simulink library "AddOn_Lib_TTC580_CCP"  (R2021a)
settings: Solver=VariableStepAuto  StartTime=0.0  StopTime=10.0  RelTol=1e-3
PreLoadFcn:
  | addpath(genpath(fileparts(which('AddOn_Lib_TTC580_CCP'))));
  | try
  | addpath([fileparts(which('AddOn_Lib_TTC580_CCP')),'\..\CustomClasses']);
  | catch
  | warning('AddOn_Lib_TTC580: add path to CustomClasses manually');
  | end
undefined symbols (not defined in the file): IO_Blk_Lib_TTC500, MainDlg_basic, MainDlg_CCP_J1939_
(part 3 of 3)

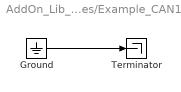
== system AddOn_Lib_TTC580_CCP/Examples/Example_CAN1 ==
  Ground : Ground
  Terminator : Terminator
  wires:
  Ground/1 -> Terminator/1

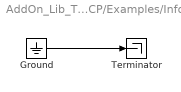
== system AddOn_Lib_TTC580_CCP/Examples/Info ==
  Ground : Ground
  Terminator : Terminator
  wires:
  Ground/1 -> Terminator/1

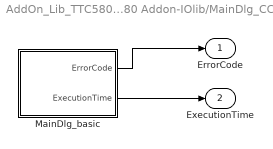
== system AddOn_Lib_TTC580_CCP/System  Blocks TTC580 Addon-IOlib/MainDlg_CCP ==
  MainDlg_basic : Subsystem  Priority=-2147483646  LoadFcn=|  mask(MainDlg_basic_Code){SampleTime=-1, ttlib=IO_Blk_Lib_TTC500, ttDescription=MainDlg_basic, tt_iolib_version=0.25, baudrate_CAN0=baudrate_CAN0, tseg1_CAN0=tseg1_CAN0, tseg2_CAN0=tseg2_CAN0, sjw_CAN0=sjw_CAN0, brp_CAN0=brp_CAN0, baudrate_CAN1=baudrate_CAN1, tseg1_CAN1=tseg1_CAN1, tseg2_CAN1=tseg2_CAN1, sjw_CAN1=sjw_CAN1, brp_CAN1=brp_CAN1, baudrate_CAN2=baudrate_CAN2, tseg1_CAN2=tseg1_CAN2, tseg2_CAN2=tseg2_CAN2, sjw_CAN2=sjw_CAN2, brp_CAN2=brp_CAN2, baudrate_CAN3=baudrate_CAN3, baudrate_CAN4=baudrate_CAN4, baudrate_CAN5=baudrate_CAN5, baudrate_CAN6=baudrate_CAN6, tseg1=tseg1, tseg2=tseg2, sjw=sjw, Duration_ms=Duration_ms, glitch_filter_time=glitch_filter_time, watchdog_window_size=watchdog_window_size, watchdog_reset_behavior=watchdog_reset_behavior, brp=brp, Major_Number=Major_Number, Minor_Number=Minor_Number, Revison_Number=Revison_Number, Node_Number=Node_Number, Enable_Reset_by_TTCDownloader=Enable_Reset_by_TTCDownloader, Enable_CCP=Enable_CCP, CRO_ID=CRO_ID, DTO_ID=DTO_ID, CCP_Station_Addr=CCP_Station_Addr, CCP_Station_ID=CCP_Station_ID, CPP_channel=CPP_channel, CPP_id_format=CPP_id_format, bEnable_DAQ0=bEnable_DAQ0, bEnable_DAQ1_2=bEnable_DAQ1_2, ODT_total=ODT_total, bEnable_ErrorCBAction=bEnable_ErrorCBAction, bDIAG_ERR_DISABLE_SSW0=bDIAG_ERR_DISABLE_SSW0, bDIAG_ERR_DISABLE_SSW1=bDIAG_ERR_DISABLE_SSW1, bDIAG_ERR_DISABLE_SSW2=bDIAG_ERR_DISABLE_SSW2, bFlashOverEthernet=bFlashOverEthernet}
      | try
      | %
      | %Upgrade Information - standard BEGIN
      | new_color = 'blue';
      | new_ver = '0.25';
      | act_ver = get_param(gcb,'tt_iolib_version');
      | if not(strcmp(act_ver,new_ver))
      |     disp(['Upgrade block: ',gcb,char(10),'       Version: ',act_ver,' to ',new_ver]);
      |     %switch - case for specific upgrade information e.g. additional parameter required 
      |     %Change appearance and version information
      |     set_param(gcb,'ForegroundColor',new_color);
      |     set_param(gcb,'tt_iolib_version',new_ver);
      | end
      | %Upgrade Information - standard END
      | catch
      | %Standard catch section BEGIN
      | errordlg('An error occurred in a callback of the TTC580-BlockLib. Please open the Diagnostic Viewer for further details');
      | disp(' ');
      | disp('------------------------------------------------------------');
      | disp('An error occurred in a callback of the TTC580-BlockLib.');
      | disp(['Please check the parameters in the mask of ',gcb]);
      | disp('If you do not encounter any violations, then please '); 
      | disp('copy the following lines and report this to support@ttcontrol.com ');
      | disp('<< begin of error message dump >>');
      | disp(['Version of TTC580-BlockLib: ', get_param(gcb,'tt_iolib_version')]);
      | disp(get_param(gcb,'ttDescription'));
      | disp(gcb);
      | x=lasterror;disp(x.message);
      | disp(get_param(gcb,'MaskValues'));
      | disp(version);
      | disp(computer);
      | disp('<< end of error message dump >>');
      | disp('------------------------------------------------------------');
      | disp(' ');
      | %Standard catch section END
      | end
      mask help:
      | Block representing the handler for main environment-settings of the applications to be run on a TTC580.
      | Generation of <model>_main.c
      mask init:
      | %
      settings: CopyFcn=%deleted
      mask Help: No further help available for this block
      mask Callback baudrate_CAN0: %
      mask Callback tseg1_CAN0: %
      mask Callback tseg2_CAN0: %
      mask Callback sjw_CAN0: %
      mask Callback brp_CAN0: %
      mask Callback baudrate_CAN1: %
      mask Callback tseg1_CAN1: %
      mask Callback tseg2_CAN1: %
      mask Callback sjw_CAN1: %
      mask Callback brp_CAN1: %
      mask Callback baudrate_CAN2: %
      mask Callback tseg1_CAN2: %
      mask Callback tseg2_CAN2: %
      mask Callback sjw_CAN2: %
      mask Callback brp_CAN2: %
      mask Callback baudrate_CAN3: %
      mask Callback baudrate_CAN4: %
      mask Callback baudrate_CAN5: %
      mask Callback baudrate_CAN6: %
      mask Callback tseg1: %
      mask Callback tseg2: %
      mask Callback sjw: %
      mask Callback Duration_ms: %
      mask Callback glitch_filter_time: %
      mask Callback watchdog_window_size: %
      mask Callback watchdog_reset_behavior: %
      mask Callback brp: %
      mask Callback Major_Number: %
      mask Callback Minor_Number: %
      mask Callback Revison_Number: %
      mask Callback Node_Number: %
      mask Callback Enable_Reset_by_TTCDownloader: %
      mask Callback Enable_CCP: %
      mask Callback CRO_ID: %
      mask Callback DTO_ID: %
      mask Callback CCP_Station_Addr: %
      mask Callback CCP_Station_ID: %
      mask Callback CPP_channel: %
      mask Callback CPP_id_format: %
      mask Callback bEnable_DAQ0: %
      mask Callback bEnable_DAQ1_2: %
      mask Callback ODT_total: %
      mask Callback bEnable_ErrorCBAction: %
      mask Callback bDIAG_ERR_DISABLE_SSW0: %
      mask Callback bDIAG_ERR_DISABLE_SSW1: %
      mask Callback bDIAG_ERR_DISABLE_SSW2: %
      mask Callback bFlashOverEthernet:
      | try
      | s_ParameterDecision = 'bFlashOverEthernet'; %Deside on this parameter
      | c_ValuesDecision={'on'}; %Positive DescitionValues
      | s_ParameterInvisible = 'Enable_Reset_by_TTCDownloader'; %Make this invisible
      | %trim
      | if ischar(s_ParameterInvisible)%if secttion for compatibility reasons of template
      |     cs_ParameterInvisible = {s_ParameterInvisible};
      | else
      |     cs_ParameterInvisible = s_ParameterInvisible;
      | end
      | s_ParameterDecision = strtrim(s_ParameterDecision);
      | c_ValuesDecision = strtrim(c_ValuesDecision);
      | for j=1:length(cs_ParameterInvisible)
      |   s_ParameterInvisible = strtrim(cs_ParameterInvisible{j});
      |   c_MaskVisibilities=get_param(gcb,'MaskVisibilities');
      |   %check consistency
      |   idx=strmatch(s_ParameterInvisible,get_param(gcb,'MaskNames'),'exact');
      |   c_MaskVisibilities{idx}='on'; %default
      |     for i = 1: length(c_ValuesDecision)
      |         if ~isempty(strmatch(get_param(gcb, s_ParameterDecision), c_ValuesDecision{i},'exact'))
      |            c_MaskVisibilities{idx}='off';
      |         end
      |     end
      |   set_param(gcb,'MaskVisibilities',c_MaskVisibilities);
      | end
      | catch
      | %Standard catch section BEGIN
      | errordlg('An error occurred in a callback of the TTC580-BlockLib. Please open the Diagnostic Viewer for further details');
      | disp(' ');
      | disp('------------------------------------------------------------');
      | disp('An error occurred in a callback of the TTC580-BlockLib.');
      | disp(['Please check the parameters in the mask of ',gcb]);
      | disp('If you do not encounter any violations, then please ');
      | disp('copy the following lines and report this to support@ttcontrol.com ');
      | disp('<< begin of error message dump >>');
      | disp(['Version of TTC580-BlockLib: ', get_param(gcb,'tt_iolib_version')]);
      | disp(get_param(gcb,'ttDescription'));
      | disp(gcb);
      | x=lasterror;disp(x.message);
      | disp(get_param(gcb,'MaskValues'));
      | disp(version);
      | disp(computer);
      | disp('<< end of error message dump >>');
      | disp('------------------------------------------------------------');
      | disp(' ');
      | %Standard catch section END
      | end
  ErrorCode : Outport  VectorParamsAs1DForOutWhenUnconnected=off
  ExecutionTime : Outport  Port=2  VectorParamsAs1DForOutWhenUnconnected=off
  wires:
  MainDlg_basic/2(ExecutionTime) -> ExecutionTime/1
  MainDlg_basic/1(ErrorCode) -> ErrorCode/1

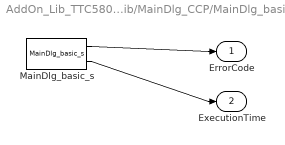
== system AddOn_Lib_TTC580_CCP/System  Blocks TTC580 Addon-IOlib/MainDlg_CCP/MainDlg_basic ==
  MainDlg_basic_s : S-Function  FunctionName=MainDlg_basic_s  Parameters=SampleTime,baudrate_CAN0,tseg1_CAN0,tseg2_CAN0,sjw_CAN0,brp_CAN0,baudrate_CAN1,tseg1_CAN1,tseg2_CAN1,sjw_CAN1,brp_CAN1,baudrate_CAN2,tseg1_CAN2,tseg2_CAN2,sjw_CAN2,brp_CAN2,baudrate_CAN3,baudrate_CAN4,baudrate_CAN5,baudrate_CAN6,tseg1,tseg2,sjw,Duration_ms,glitch_filter_time,watchdog_window_size,watchdog_reset_behavior,brp,Major_Number,Minor_Number,Revison_Number,Node_Number,Enable_Reset_by_TTCDownloader,Enable_CCP,CRO_ID,DTO_ID,CCP_Station_Addr,CCP_Station_ID,CPP_channel,CPP_id_format,bEnable_DAQ0,bEnable_DAQ1_2,ODT_total,bEnable_ErrorCBAction,bDIAG_ERR_DISABLE_SSW0,bDIAG_ERR_DISABLE_SSW1,bDIAG_ERR_DISABLE_SSW2,bFlashOverEthernet  SFunctionDeploymentMode=off  EnableBusSupport=off
  ErrorCode : Outport
  ExecutionTime : Outport  Port=2
  wires:
  MainDlg_basic_s/2 -> ExecutionTime/1
  MainDlg_basic_s/1 -> ErrorCode/1
